simulink model "lab11_simulink"  (R2023a)
settings: Solver=VariableStepAuto  StartTime=0.0  StopTime=10.0  RelTol=1e-3
settings Model: Creator=laura  LastModifiedBy=mluser

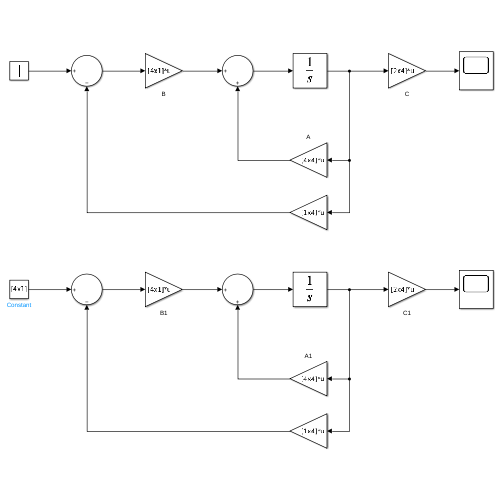
[thumbnail: Simulink's stored preview of the top-level diagram]
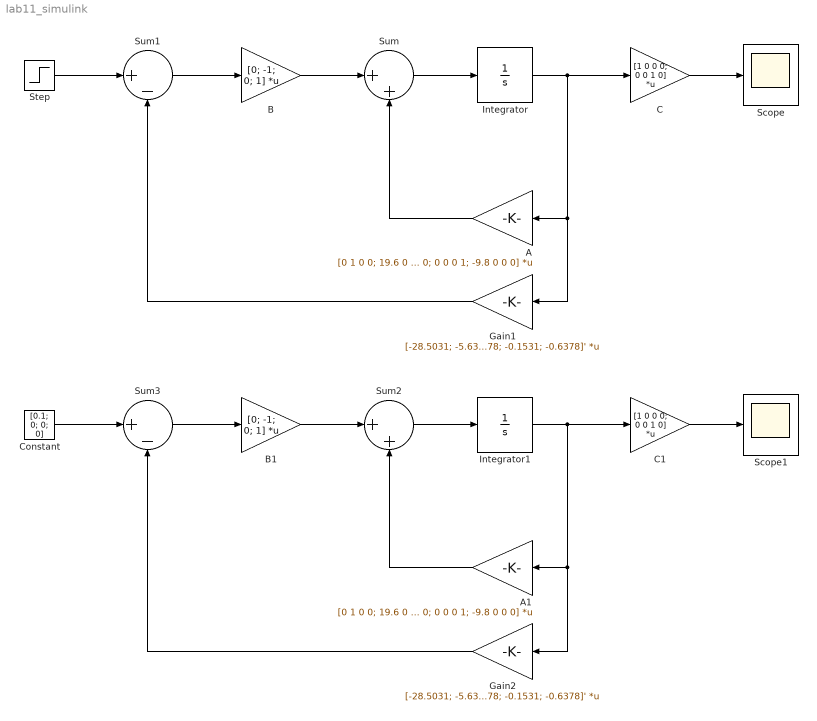
== system lab11_simulink ==
  A : Gain  Gain=[0 1 0 0; 19.6 0 0 0; 0 0 0 1; -9.8 0 0 0]  Multiplication=Matrix(K*u)
  A1 : Gain  Gain=[0 1 0 0; 19.6 0 0 0; 0 0 0 1; -9.8 0 0 0]  Multiplication=Matrix(K*u)
  B : Gain  Gain=[0; -1; 0; 1]  Multiplication=Matrix(K*u)
  B1 : Gain  Gain=[0; -1; 0; 1]  Multiplication=Matrix(K*u)
  C : Gain  Gain=[1 0 0 0; 0 0 1 0]  Multiplication=Matrix(K*u)
  C1 : Gain  Gain=[1 0 0 0; 0 0 1 0]  Multiplication=Matrix(K*u)
  Constant : Constant  Value=[0.1; 0; 0; 0]
  Gain1 : Gain  Gain=[-28.5031; -5.6378; -0.1531; -0.6378]'  Multiplication=Matrix(K*u)
  Gain2 : Gain  Gain=[-28.5031; -5.6378; -0.1531; -0.6378]'  Multiplication=Matrix(K*u)
  Integrator : Integrator
  Integrator1 : Integrator
  Scope : Scope
  Scope1 : Scope
  Step : Step  Time=0.2  Before=1  After=0  SampleTime=0
  Sum : Sum  Inputs=|++
  Sum1 : Sum  Inputs=|+-
  Sum2 : Sum  Inputs=|++
  Sum3 : Sum  Inputs=|+-
  wires:
  B/1 -> Sum/1
  Sum/1 -> Integrator/1
  Integrator/1 -> Gain1/1, A/1, C/1
  A/1 -> Sum/2
  C/1 -> Scope/1
  Sum1/1 -> B/1
  Gain1/1 -> Sum1/2
  Step/1 -> Sum1/1
  Constant/1 -> Sum3/1
  Gain2/1 -> Sum3/2
  B1/1 -> Sum2/1
  A1/1 -> Sum2/2
  Sum2/1 -> Integrator1/1
  Sum3/1 -> B1/1
  C1/1 -> Scope1/1
  Integrator1/1 -> Gain2/1, A1/1, C1/1
